simulink model "vehicle_14dof_4wis_4wid"  (R2022b)
settings: Solver=ode15s  StartTime=0  StopTime=5  MaxStep=0.005  RelTol=1e-4  AbsTol=1e-6
model workspace (MAT data in the model file):
  p_14dof.M = 1500
  p_14dof.m_s = 1350
  p_14dof.m_uf = 35
  p_14dof.m_ur = 40
  p_14dof.a = 1.2
  p_14dof.b = 1.3
  p_14dof.L = 2.5
  p_14dof.B_f = 1.52
  p_14dof.B_r = 1.52
  p_14dof.B_sf = 1.2
  p_14dof.B_sr = 1.2
  p_14dof.h_g = 0.55
  p_14dof.h_rcf = 0.08
  p_14dof.h_rcr = 0.1
  p_14dof.d_roll = 0.46
  p_14dof.d_pitch = 0.46
  p_14dof.I_x = 450
  p_14dof.I_y = 2200
  p_14dof.I_z = 2500
  p_14dof.I_w = 1.5
  p_14dof.I_xz = 0
  p_14dof.K_s1_f = 22000
  p_14dof.K_s2_f = 4000000
  p_14dof.C_s1_f = 2800
  p_14dof.C_s2_f = 800
  p_14dof.xi_reb_comp = 2.75
  p_14dof.K_d_susp = 15
  p_14dof.K_s1_r = 20000
  p_14dof.K_s2_r = 3500000
  p_14dof.C_s1_r = 2500
  p_14dof.C_s2_r = 700
  p_14dof.K_t = 210000
  p_14dof.C_t = 5000
  p_14dof.r_w = 0.31
  p_14dof.B_y = 8
  p_14dof.C_y = 1.3
  p_14dof.D_y = 4200
  p_14dof.E_y = -1.6
  p_14dof.n_Fz = 0.8
  p_14dof.B_x = 12
  p_14dof.C_x = 1.65
  p_14dof.D_x = 4200
  p_14dof.E_x = -1.2
  p_14dof.Fz0 = 4000
  p_14dof.mu_x = 1.05
  p_14dof.mu_y = 1.05
  p_14dof.sigma_x = 0.3
  p_14dof.sigma_y = 0.6
  p_14dof.T_m_max = 300
  p_14dof.T_m_regen_max = 100
  p_14dof.T_m_rated = 150
  p_14dof.P_m_rated = 30000
  p_14dof.omega_m_max = 1200
  p_14dof.d_brake_master = 0.0222
  p_14dof.i_brake_pedal = 4.1
  p_14dof.eta_brake_pedal = 0.86
  p_14dof.k_brake_boost = 3.5
  p_14dof.d_brake_caliper_f = 0.04789
  p_14dof.d_brake_caliper_r = 0.0329
  p_14dof.eta_brake_caliper = 0.85
  p_14dof.mu_brake_pad = 0.35
  p_14dof.r_brake_disc_f = 0.105
  p_14dof.r_brake_disc_r = 0.113
  p_14dof.F_pedal_max = 300
  p_14dof.i_st = 18
  p_14dof.g = 9.81
  p_14dof.f_roll = 0.015
  p_14dof.rho_air = 1.225
  p_14dof.C_d = 0.3
  p_14dof.A_f = 2.2
  p_14dof.slope_max_deg = 30
  p_14dof.slope_max_rad = 0.523598775598
  p_14dof.slope_max = 0.57735026919
  p_14dof.eps_v = 0.2
  p_14dof.eps_gnd = 0.001
  p_14dof.inv_tau_min = 5
  p_14dof.T_ramp = 1
  p_14dof.vx0 = 8.33333333333
  p_14dof.Kp_speed = 1000
  p_14dof.Kp_brake = 0.75
  p_14dof.brake_deadband = 0.03
  p_14dof.brake_cruise_deadband = 0.5
  p_14dof.beta_brk_auto_max = 0.6
  p_14dof.use_dyn_load_transfer = 0
  p_14dof.ctrl.mode = 3
  p_14dof.ctrl.Kp_speed = 1000
  p_14dof.ctrl.Kp_brake = 0.05
  p_14dof.ctrl.K_blend = 5
  p_14dof.ctrl.kappa_thr = 0.15
  p_14dof.ctrl.K_asr_blend = 10
  p_14dof.ctrl.Kp_yaw = 500
  p_14dof.ctrl.Ki_yaw = 100
  p_14dof.ctrl.yaw_int_max = 200
  p_14dof.ctrl.tau_tvc = 0.05
  p_14dof.ctrl.yaw_split_front = 0.5
  p_14dof.vx0_save = 8.33333333333
  p_14dof.vx0_save2 = 8.33333333333
settings Model: Creator=admin  LastModifiedBy=admin

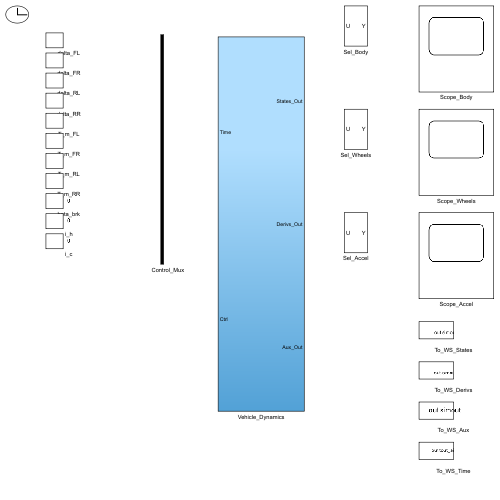
[thumbnail: Simulink's stored preview of the top-level diagram]
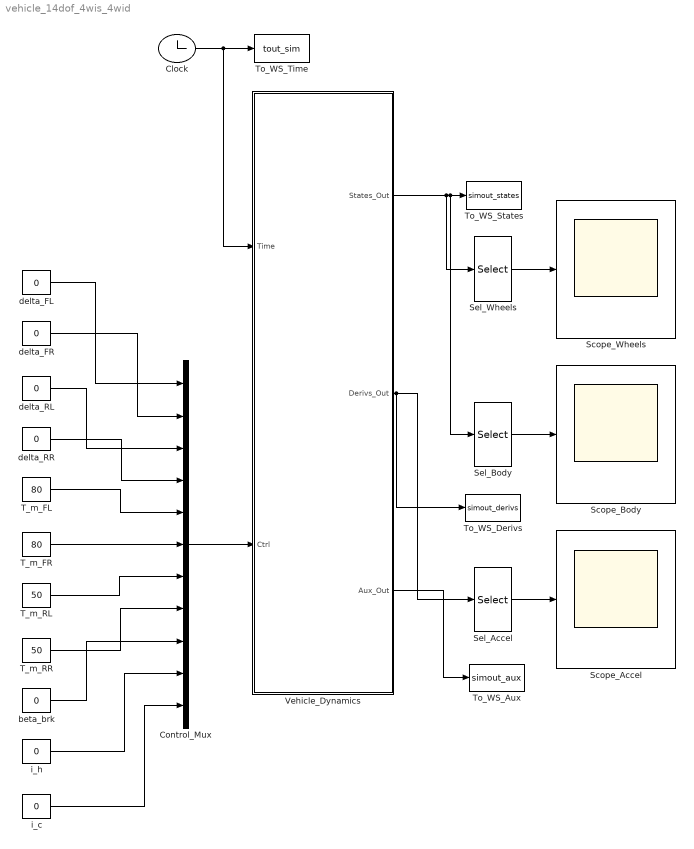
== system vehicle_14dof_4wis_4wid ==
  Clock : Clock
  Control_Mux : Mux  Inputs=11
  Scope_Accel : Scope
  Scope_Body : Scope
  Scope_Wheels : Scope
  Sel_Accel : Selector  InputPortWidth=29  IndexOptions=Index vector (dialog)  Indices=[1 2 4 6 8 9]  OutputSizes=6
  Sel_Body : Selector  InputPortWidth=29  IndexOptions=Index vector (dialog)  Indices=[1 2 3 5 7 9]  OutputSizes=6
  Sel_Wheels : Selector  InputPortWidth=29  IndexOptions=Index vector (dialog)  Indices=[10 11 12 13 14 15 16 17]  OutputSizes=8
  T_m_FL : Constant  Value=80
  T_m_FR : Constant  Value=80
  T_m_RL : Constant  Value=50
  T_m_RR : Constant  Value=50
  To_WS_Aux : ToWorkspace  VariableName=simout_aux  SampleTime=-1
  To_WS_Derivs : ToWorkspace  VariableName=simout_derivs  SampleTime=-1
  To_WS_States : ToWorkspace  VariableName=simout_states  SampleTime=-1
  To_WS_Time : ToWorkspace  VariableName=tout_sim  SampleTime=-1
  Vehicle_Dynamics : Subsystem
  beta_brk : Constant  Value=0
  delta_FL : Constant  Value=0
  delta_FR : Constant  Value=0
  delta_RL : Constant  Value=0
  delta_RR : Constant  Value=0
  i_c : Constant  Value=0
  i_h : Constant  Value=0
  wires:
  Clock/1 -> Vehicle_Dynamics/1(Time), To_WS_Time/1
  T_m_FR/1 -> Control_Mux/6
  T_m_RL/1 -> Control_Mux/7
  delta_FL/1 -> Control_Mux/1
  Control_Mux/1 -> Vehicle_Dynamics/2(Ctrl)
  delta_RR/1 -> Control_Mux/4
  delta_FR/1 -> Control_Mux/2
  T_m_FL/1 -> Control_Mux/5
  delta_RL/1 -> Control_Mux/3
  T_m_RR/1 -> Control_Mux/8
  beta_brk/1 -> Control_Mux/9
  i_c/1 -> Control_Mux/11
  i_h/1 -> Control_Mux/10
  Vehicle_Dynamics/1(States_Out) -> To_WS_States/1, Sel_Body/1, Sel_Wheels/1
  Vehicle_Dynamics/2(Derivs_Out) -> Sel_Accel/1, To_WS_Derivs/1
  Vehicle_Dynamics/3(Aux_Out) -> To_WS_Aux/1
  Sel_Wheels/1 -> Scope_Wheels/1
  Sel_Body/1 -> Scope_Body/1
  Sel_Accel/1 -> Scope_Accel/1

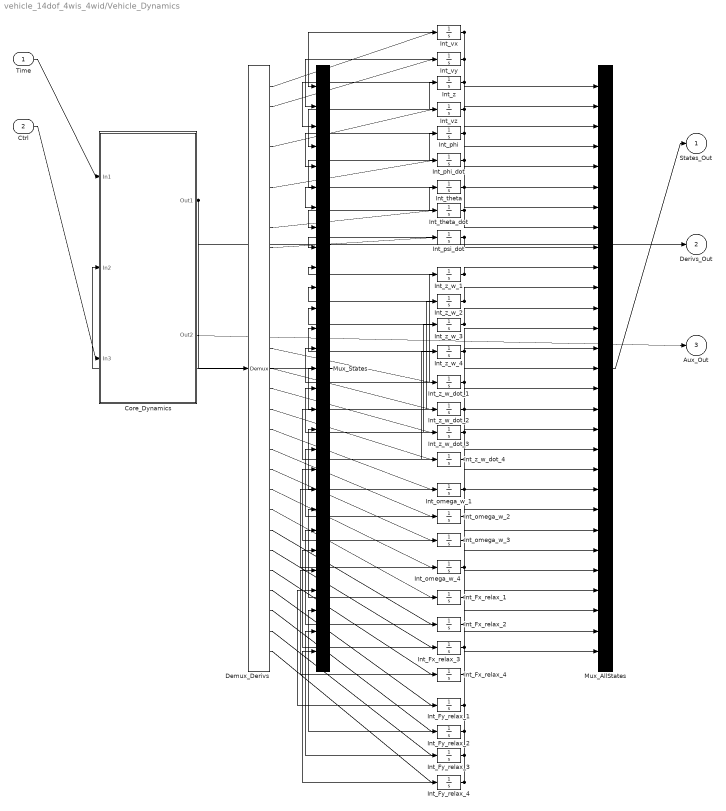
== system vehicle_14dof_4wis_4wid/Vehicle_Dynamics ==
  Time : Inport
  Ctrl : Inport  Port=2  PortDimensions=11
  Core_Dynamics : Subsystem
  Demux_Derivs : Demux  Outputs=29
  Int_Fx_relax_{1..4} (4 alike) : Integrator
  Int_Fy_relax_{1..4} (4 alike) : Integrator
  Int_omega_w_{1..4} (4 alike) : Integrator  InitialCondition=26.8817
  Int_phi : Integrator
  Int_phi_dot : Integrator
  Int_psi_dot : Integrator
  Int_theta : Integrator
  Int_theta_dot : Integrator
  Int_vx : Integrator  InitialCondition=8.3333
  Int_vy : Integrator
  Int_vz : Integrator
  Int_z : Integrator  InitialCondition=-0.017518
  Int_z_w_1 : Integrator  InitialCondition=-0.018032
  Int_z_w_2 : Integrator  InitialCondition=-0.018032
  Int_z_w_3 : Integrator  InitialCondition=-0.017004
  Int_z_w_4 : Integrator  InitialCondition=-0.017004
  Int_z_w_dot_{1..4} (4 alike) : Integrator
  Mux_AllStates : Mux  Inputs=29
  Mux_States : Mux  Inputs=29
  States_Out : Outport  PortDimensions=29
  Derivs_Out : Outport  Port=2  PortDimensions=29
  Aux_Out : Outport  Port=3  PortDimensions=52
  wires:
  Int_vx/1 -> Mux_States/1, Mux_AllStates/1
  Int_vy/1 -> Mux_States/2, Mux_AllStates/2
  Int_z/1 -> Mux_States/3, Mux_AllStates/3
  Int_vz/1 -> Mux_States/4, Int_z/1, Mux_AllStates/4
  Int_phi/1 -> Mux_States/5, Mux_AllStates/5
  Int_phi_dot/1 -> Mux_States/6, Int_phi/1, Mux_AllStates/6
  Int_theta/1 -> Mux_States/7, Mux_AllStates/7
  Int_theta_dot/1 -> Mux_States/8, Int_theta/1, Mux_AllStates/8
  Int_psi_dot/1 -> Mux_States/9, Mux_AllStates/9
  Int_z_w_1/1 -> Mux_States/10, Mux_AllStates/10
  Int_z_w_2/1 -> Mux_States/11, Mux_AllStates/11
  Int_z_w_3/1 -> Mux_States/12, Mux_AllStates/12
  Int_z_w_4/1 -> Mux_States/13, Mux_AllStates/13
  Int_z_w_dot_1/1 -> Mux_States/14, Int_z_w_1/1, Mux_AllStates/14
  Int_z_w_dot_2/1 -> Mux_States/15, Int_z_w_2/1, Mux_AllStates/15
  Int_z_w_dot_3/1 -> Mux_States/16, Int_z_w_3/1, Mux_AllStates/16
  Int_z_w_dot_4/1 -> Mux_States/17, Int_z_w_4/1, Mux_AllStates/17
  Int_omega_w_1/1 -> Mux_States/18, Mux_AllStates/18
  Int_omega_w_2/1 -> Mux_States/19, Mux_AllStates/19
  Int_omega_w_3/1 -> Mux_States/20, Mux_AllStates/20
  Int_omega_w_4/1 -> Mux_States/21, Mux_AllStates/21
  Int_Fx_relax_1/1 -> Mux_States/22, Mux_AllStates/22
  Int_Fx_relax_2/1 -> Mux_States/23, Mux_AllStates/23
  Int_Fx_relax_3/1 -> Mux_States/24, Mux_AllStates/24
  Int_Fx_relax_4/1 -> Mux_States/25, Mux_AllStates/25
  Int_Fy_relax_1/1 -> Mux_States/26, Mux_AllStates/26
  Int_Fy_relax_2/1 -> Mux_States/27, Mux_AllStates/27
  Int_Fy_relax_3/1 -> Mux_States/28, Mux_AllStates/28
  Int_Fy_relax_4/1 -> Mux_States/29, Mux_AllStates/29
  Time/1 -> Core_Dynamics/1(In1)
  Mux_States/1 -> Core_Dynamics/2(In2)
  Ctrl/1 -> Core_Dynamics/3(In3)
  Core_Dynamics/1(Out1) -> Demux_Derivs/1, Derivs_Out/1
  Demux_Derivs/1 -> Int_vx/1
  Demux_Derivs/2 -> Int_vy/1
  Demux_Derivs/4 -> Int_vz/1
  Demux_Derivs/6 -> Int_phi_dot/1
  Demux_Derivs/8 -> Int_theta_dot/1
  Demux_Derivs/9 -> Int_psi_dot/1
  Demux_Derivs/14 -> Int_z_w_dot_1/1
  Demux_Derivs/15 -> Int_z_w_dot_2/1
  Demux_Derivs/16 -> Int_z_w_dot_3/1
  Demux_Derivs/17 -> Int_z_w_dot_4/1
  Demux_Derivs/18 -> Int_omega_w_1/1
  Demux_Derivs/19 -> Int_omega_w_2/1
  Demux_Derivs/20 -> Int_omega_w_3/1
  Demux_Derivs/21 -> Int_omega_w_4/1
  Demux_Derivs/22 -> Int_Fx_relax_1/1
  Demux_Derivs/23 -> Int_Fx_relax_2/1
  Demux_Derivs/24 -> Int_Fx_relax_3/1
  Demux_Derivs/25 -> Int_Fx_relax_4/1
  Demux_Derivs/26 -> Int_Fy_relax_1/1
  Demux_Derivs/27 -> Int_Fy_relax_2/1
  Demux_Derivs/28 -> Int_Fy_relax_3/1
  Demux_Derivs/29 -> Int_Fy_relax_4/1
  Mux_AllStates/1 -> States_Out/1
  Core_Dynamics/2(Out2) -> Aux_Out/1

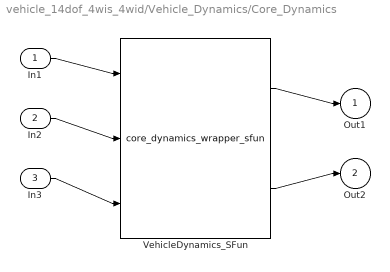
== system vehicle_14dof_4wis_4wid/Vehicle_Dynamics/Core_Dynamics ==
  In1 : Inport
  In2 : Inport  Port=2  PortDimensions=29
  In3 : Inport  Port=3  PortDimensions=11
  VehicleDynamics_SFun : M-S-Function  FunctionName=core_dynamics_wrapper_sfun  Parameters=p_14dof
  Out1 : Outport  PortDimensions=29
  Out2 : Outport  Port=2  PortDimensions=52
  wires:
  In1/1 -> VehicleDynamics_SFun/1
  In2/1 -> VehicleDynamics_SFun/2
  In3/1 -> VehicleDynamics_SFun/3
  VehicleDynamics_SFun/1 -> Out1/1
  VehicleDynamics_SFun/2 -> Out2/1
